simulink model "speaker-model"  (R2021b)
settings: Solver=VariableStepAuto  StartTime=0.0  StopTime=4.5  RelTol=1e-3
model workspace (MAT data in the model file):
  Ms = 8e-06
  Re = 31.75
  Rms = 0.09
undefined symbols (not defined in the file): High
libraries: dspsigops x3, dspsrcs4 x1
settings Model: Creator=Anush  LastModifiedBy=Anush

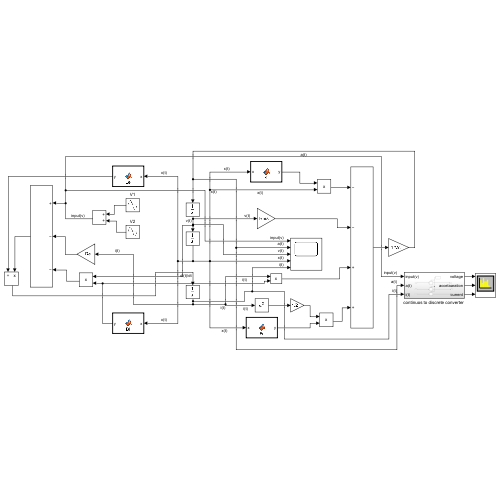
[thumbnail: Simulink's stored preview of the top-level diagram]
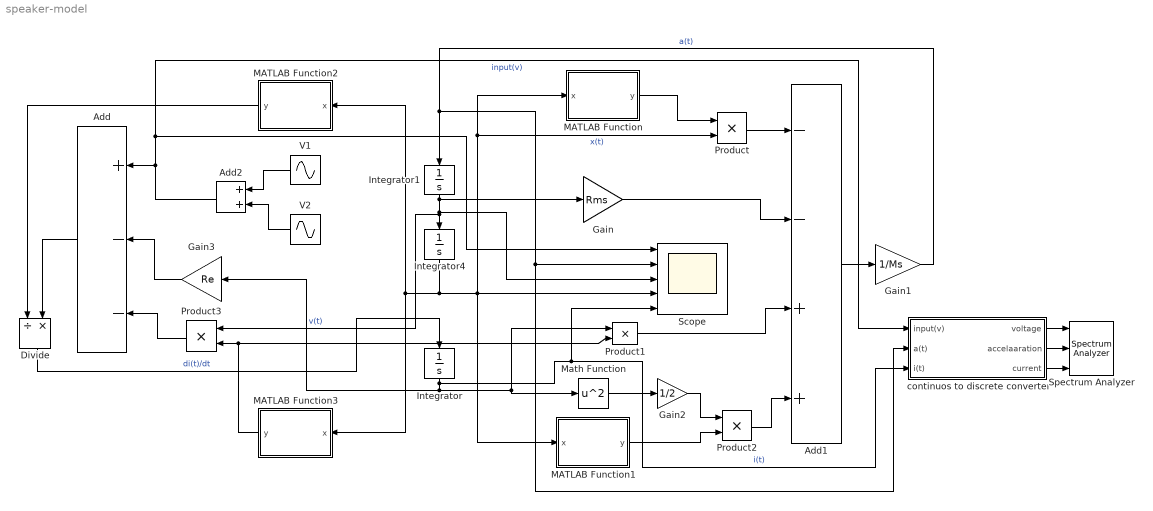
== system speaker-model ==
  Add : Sum  Inputs=+--
  Add1 : Sum  Inputs=--++
  Add2 : Sum
  Divide : Product  Inputs=/*
  Gain : Gain  Gain=Rms
  Gain1 : Gain  Gain=1/Ms
  Gain2 : Gain  Gain=1/2
  Gain3 : Gain  Gain=Re
  Integrator : Integrator
  Integrator1 : Integrator
  Integrator4 : Integrator
  MATLAB Function : MATLAB Function  TreatAsAtomicUnit=on
  MATLAB Function1 : MATLAB Function  TreatAsAtomicUnit=on
  MATLAB Function2 : MATLAB Function  TreatAsAtomicUnit=on
  MATLAB Function3 : MATLAB Function  TreatAsAtomicUnit=on
  Math Function : Math  Operator=square  SaturateOnIntegerOverflow=on
  Product{,1..3} (4 alike) : Product
  Scope : Scope  NumInputPorts=5
  Spectrum Analyzer : SpectrumAnalyzer  NumInputPorts=3
  V1 : Sin  Amplitude=0.944  Frequency=2*pi*541  SampleTime=0
  V2 : Sin  Amplitude=0.237  Frequency=2*pi*5447  SampleTime=0
  "continuos to discrete converter " : Subsystem
  wires:
  Integrator/1 -> Scope/5, "continuos to discrete converter "/3(i(t)), Gain3/1, Product1/1, Math Function/1  "i(t)"
  Integrator1/1 -> Scope/3, Product3/1, Integrator4/1, Gain/1  "v(t)"
  Integrator4/1 -> Scope/4, MATLAB Function1/1(x), MATLAB Function/1(x), Product/2, MATLAB Function3/1(x), MATLAB Function2/1(x)  "x(t)"
  Gain1/1 -> Scope/2, "continuos to discrete converter "/2(a(t)), Integrator1/1  "a(t)"
  Divide/1 -> Integrator/1  "di(t)/dt"
  Add1/1 -> Gain1/1
  Gain/1 -> Add1/2
  MATLAB Function/1(y) -> Product/1
  Product/1 -> Add1/1
  Product1/1 -> Add1/3
  Math Function/1 -> Gain2/1
  Gain2/1 -> Product2/1
  MATLAB Function1/1(y) -> Product2/2
  Product2/1 -> Add1/4
  V2/1 -> Add2/2
  V1/1 -> Add2/1
  Add2/1 -> Scope/1, "continuos to discrete converter "/1(input(v)), Add/1  "input(v)"
  Gain3/1 -> Add/2
  MATLAB Function3/1(y) -> Product3/2, Product1/2
  Product3/1 -> Add/3
  Add/1 -> Divide/2
  MATLAB Function2/1(y) -> Divide/1
  "continuos to discrete converter "/3(current) -> Spectrum Analyzer/3
  "continuos to discrete converter "/2(accelaaration) -> Spectrum Analyzer/2
  "continuos to discrete converter "/1(voltage) -> Spectrum Analyzer/1

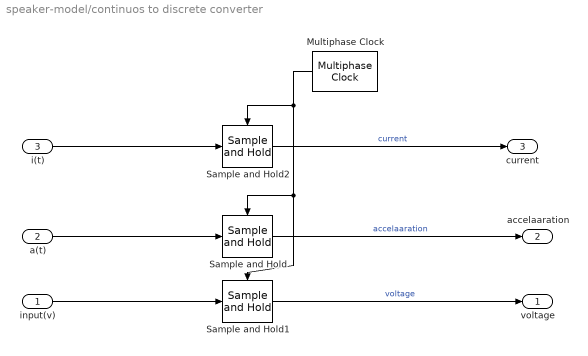
== system speaker-model/continuos to discrete converter  ==
  input(v) : Inport
  a(t) : Inport  Port=2
  i(t) : Inport  Port=3
  Multiphase Clock : dspsrcs4/Multiphase Clock  ClkFreq=20000  NumPhases=4  StartPhase=1  DutyCycle=3  ActiveLevel=High (1)  DataType=Logical
      settings: SourceProductBaseCode=DS
  Sample and Hold : dspsigops/Sample and Hold  trig=Rising edge  initCond=0  latchinput=off
  Sample and Hold1 : dspsigops/Sample and Hold  trig=Rising edge  initCond=0  latchinput=off
  Sample and Hold2 : dspsigops/Sample and Hold  trig=Rising edge  initCond=0  latchinput=off
  voltage : Outport
  accelaaration : Outport  Port=2
  current : Outport  Port=3
  wires:
  input(v)/1 -> Sample and Hold1/1
  a(t)/1 -> Sample and Hold/1
  Multiphase Clock/1 -> Sample and Hold1/Trigger, Sample and Hold/Trigger, Sample and Hold2/Trigger
  i(t)/1 -> Sample and Hold2/1
  Sample and Hold1/1 -> voltage/1  "voltage"
  Sample and Hold2/1 -> current/1  "current"
  Sample and Hold/1 -> accelaaration/1  "accelaaration"

== matlab function speaker-model/MATLAB Function ==
  data: x input; y output
function y = K(x)

y = 41.75+(25.02*x) + (150.37*x^2)+(388.08*x^3)-(2382.67*x^4)+(74.63*x^5)+(128.09*x^6);

== matlab function speaker-model/MATLAB Function2 ==
  data: x input; y output
function y = Le(x)

y = (6.01*10^-5)-(1.46*(10^-2)*x)+(0.61*x^2) +(1.31*10^4*x^3)+ (6.52*10^6*x^4)-(5.18*10^10*x^5)-(4.42*10^13*x^6);

== matlab function speaker-model/MATLAB Function3 ==
  data: x input; y output
function y = Bl(x)

y = 0.23-(165*x)-(1.61*10^5*x^2)+ (6.49*10^8*x^3)-(5.97*10^12*x^4)+(1.06*10^15*x^5)+(2.14*10^19*x^6);

== matlab function speaker-model/MATLAB Function1 ==
  data: x input; y output
function y = Fr(x)

y = -(1.46*(10^-2))+(2*0.61*x) +(3*1.31*10^4*x^2)+ (4*6.52*10^6*x^3)-(5*5.18*10^10*x^4)-(6*4.42*10^13*x^5);
